simulink model "ej3"  (R2020b)
settings: Solver=ode4  StartTime=0.0  StopTime=30.0  FixedStep=0.05  RelTol=1e-3
settings Model: Creator=Kike  LastModifiedBy=zunt7

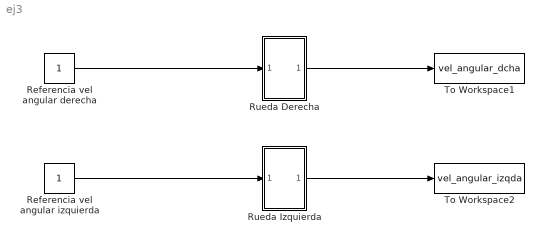
== system ej3 ==
  Referencia vel angular derecha : Constant
  Referencia vel angular izquierda : Constant
  Rueda Derecha : Subsystem
  Rueda Izquierda : Subsystem
  To Workspace1 : ToWorkspace  VariableName=vel_angular_dcha  SaveFormat=Timeseries  SampleTime=-1
  To Workspace2 : ToWorkspace  VariableName=vel_angular_izqda  SaveFormat=Timeseries  SampleTime=-1
  wires:
  Referencia vel angular derecha/1 -> Rueda Derecha/1(In1)
  Rueda Derecha/1(Out1) -> To Workspace1/1
  Rueda Izquierda/1(Out1) -> To Workspace2/1
  Referencia vel angular izquierda/1 -> Rueda Izquierda/1(In1)

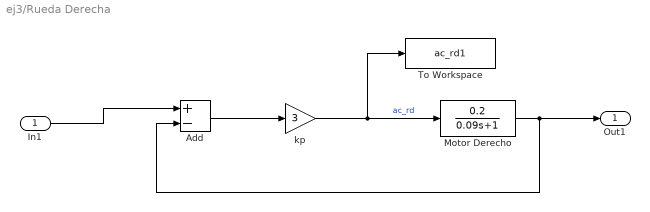
== system ej3/Rueda Derecha ==
  In1 : Inport
  Add : Sum  Inputs=+-
  Motor Derecho : TransferFcn  Numerator=[0.2]  Denominator=[0.09 1]
  To Workspace : ToWorkspace  VariableName=ac_rd1  SaveFormat=Timeseries  SampleTime=-1
  kp : Gain  Gain=3
  Out1 : Outport
  wires:
  In1/1 -> Add/1
  kp/1 -> To Workspace/1, Motor Derecho/1  "ac_rd"
  Add/1 -> kp/1
  Motor Derecho/1 -> Out1/1, Add/2

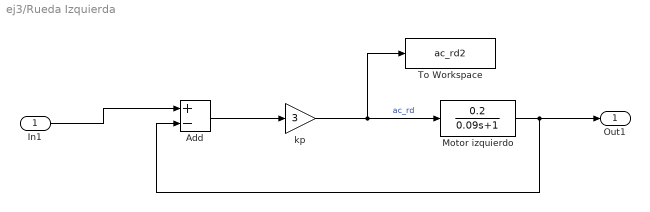
== system ej3/Rueda Izquierda ==
  In1 : Inport
  Add : Sum  Inputs=+-
  Motor izquierdo : TransferFcn  Numerator=[0.2]  Denominator=[0.09 1]
  To Workspace : ToWorkspace  VariableName=ac_rd2  SaveFormat=Timeseries  SampleTime=-1
  kp : Gain  Gain=3
  Out1 : Outport
  wires:
  In1/1 -> Add/1
  kp/1 -> To Workspace/1, Motor izquierdo/1  "ac_rd"
  Add/1 -> kp/1
  Motor izquierdo/1 -> Out1/1, Add/2
